simulink model "E3_2_B_Desequilibrio"  (R2018a)
settings: Solver=VariableStepAuto  StartTime=0.0  StopTime=1  RelTol=1e-3
libraries: powerlib x22, powerlib_meascontrol x20
settings Model: Creator=Rafael Pavan  LastModifiedBy=Rafael Pavan

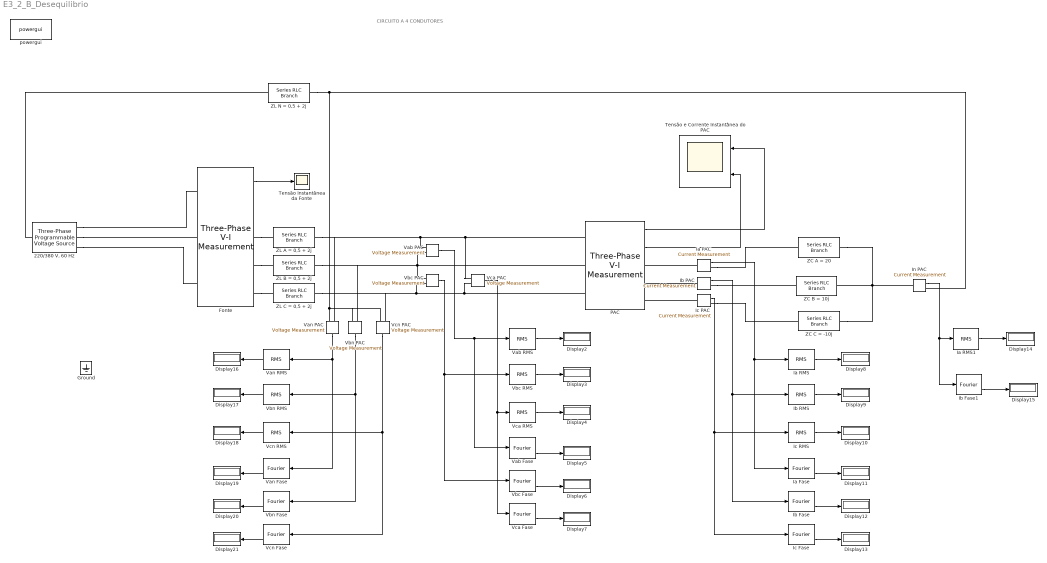
== system E3_2_B_Desequilibrio ==
  note: CIRCUITO A 4 CONDUTORES
  "220/380 V, 60 Hz" : powerlib/Electrical Sources/Three-Phase Programmable Voltage Source  PositiveSequence=[380 0 60]  VariationEntity=None  VariationType=Table of time-amplitude pairs  VariationTypeAlt=Step  VariationStep=0.5  VariationRate=10  VariationMagnitude=0.3  VariationFrequency=2  VariationTiming=[1 2]  VariationPhaseA=off  Amplitudes=[1 0.8 1.2 1.0]  TimeValues=[0 0.1 0.15 0.2]  HarmonicGeneration=off  HarmonicA=[3 0.2 -25 0]  HarmonicB=[2 0.15 35 2]  Timing="[0.05  3]"  BusType=PV  Pref=1000000000  Qref=0  Qmin=-inf  Qmax=inf
  Display{2..21} (20 alike) : Display
  Fonte : powerlib/Measurements/Three-Phase V-I Measurement  VoltageMeasurement=phase-to-phase  SetLabelV=off  LabelV=Vabc  Vpu=off  VpuLL=off  CurrentMeasurement=yes  SetLabelI=off  LabelI=Iabc  Ipu=off  Pbase=100e6  Vbase=220  OutputType=Complex  PhasorSimulation=off  PSBequivalent=0
  Ground : powerlib/Elements/Ground  LConnTagsString=a
  Ia Fase : powerlib_meascontrol/Measurements/Fourier  Freq=60  n=1  InInit=[0, 0]  Ts=0
      settings: SourceProductName=Simscape Power Systems
  Ia PAC : powerlib/Measurements/Current Measurement  PhasorSimulation=off  OutputType=Complex  PSBequivalent=0
  Ia RMS : powerlib_meascontrol/Measurements/RMS  TrueRMS=on  Freq=60  RMSInit=120  Ts=0
  Ia RMS1 : powerlib_meascontrol/Measurements/RMS  TrueRMS=on  Freq=60  RMSInit=120  Ts=0
  Ib Fase : powerlib_meascontrol/Measurements/Fourier  Freq=60  n=1  InInit=[0, 0]  Ts=0
      settings: SourceProductName=Simscape Power Systems
  Ib Fase1 : powerlib_meascontrol/Measurements/Fourier  Freq=60  n=1  InInit=[0, 0]  Ts=0
      settings: SourceProductName=Simscape Power Systems
  Ib PAC : powerlib/Measurements/Current Measurement  PhasorSimulation=off  OutputType=Complex  PSBequivalent=0
  Ib RMS : powerlib_meascontrol/Measurements/RMS  TrueRMS=on  Freq=60  RMSInit=120  Ts=0
  Ic Fase : powerlib_meascontrol/Measurements/Fourier  Freq=60  n=1  InInit=[0, 0]  Ts=0
      settings: SourceProductName=Simscape Power Systems
  Ic PAC : powerlib/Measurements/Current Measurement  PhasorSimulation=off  OutputType=Complex  PSBequivalent=0
  Ic RMS : powerlib_meascontrol/Measurements/RMS  TrueRMS=on  Freq=60  RMSInit=120  Ts=0
  In PAC : powerlib/Measurements/Current Measurement  PhasorSimulation=off  OutputType=Complex  PSBequivalent=0
  PAC : powerlib/Measurements/Three-Phase V-I Measurement  VoltageMeasurement=phase-to-phase  SetLabelV=off  LabelV=Vabc  Vpu=off  VpuLL=off  CurrentMeasurement=yes  SetLabelI=off  LabelI=Iabc  Ipu=off  Pbase=100e6  Vbase=220  OutputType=Complex  PhasorSimulation=off  PSBequivalent=0
  Tensão Instantânea da Fonte : Scope
  Tensão e Corrente Instantânea do PAC : Scope  NumInputPorts=2
  Vab Fase : powerlib_meascontrol/Measurements/Fourier  Freq=60  n=1  InInit=[0, 0]  Ts=0
      settings: SourceProductName=Simscape Power Systems
  Vab PAC : powerlib/Measurements/Voltage Measurement  PhasorSimulation=off  OutputType=Complex  PSBequivalent=0
  Vab RMS : powerlib_meascontrol/Measurements/RMS  TrueRMS=on  Freq=60  RMSInit=120  Ts=0
  Van Fase : powerlib_meascontrol/Measurements/Fourier  Freq=60  n=1  InInit=[0, 0]  Ts=0
      settings: SourceProductName=Simscape Power Systems
  Van PAC : powerlib/Measurements/Voltage Measurement  PhasorSimulation=off  OutputType=Complex  PSBequivalent=0
  Van RMS : powerlib_meascontrol/Measurements/RMS  TrueRMS=on  Freq=60  RMSInit=120  Ts=0
  Vbc Fase : powerlib_meascontrol/Measurements/Fourier  Freq=60  n=1  InInit=[0, 0]  Ts=0
      settings: SourceProductName=Simscape Power Systems
  Vbc PAC : powerlib/Measurements/Voltage Measurement  PhasorSimulation=off  OutputType=Complex  PSBequivalent=0
  Vbc RMS : powerlib_meascontrol/Measurements/RMS  TrueRMS=on  Freq=60  RMSInit=120  Ts=0
  Vbn Fase : powerlib_meascontrol/Measurements/Fourier  Freq=60  n=1  InInit=[0, 0]  Ts=0
      settings: SourceProductName=Simscape Power Systems
  Vbn PAC : powerlib/Measurements/Voltage Measurement  PhasorSimulation=off  OutputType=Complex  PSBequivalent=0
  Vbn RMS : powerlib_meascontrol/Measurements/RMS  TrueRMS=on  Freq=60  RMSInit=120  Ts=0
  Vca Fase : powerlib_meascontrol/Measurements/Fourier  Freq=60  n=1  InInit=[0, 0]  Ts=0
      settings: SourceProductName=Simscape Power Systems
  Vca PAC : powerlib/Measurements/Voltage Measurement  PhasorSimulation=off  OutputType=Complex  PSBequivalent=0
  Vca RMS : powerlib_meascontrol/Measurements/RMS  TrueRMS=on  Freq=60  RMSInit=120  Ts=0
  Vcn Fase : powerlib_meascontrol/Measurements/Fourier  Freq=60  n=1  InInit=[0, 0]  Ts=0
      settings: SourceProductName=Simscape Power Systems
  Vcn PAC : powerlib/Measurements/Voltage Measurement  PhasorSimulation=off  OutputType=Complex  PSBequivalent=0
  Vcn RMS : powerlib_meascontrol/Measurements/RMS  TrueRMS=on  Freq=60  RMSInit=120  Ts=0
  ZC A = 20 : powerlib/Elements/Series RLC Branch  LConnTagsString=__new0  RConnTagsString=__new0  BranchType=R  Resistance=20  Inductance=0  SetiL0=off  InitialCurrent=0  Capacitance=1e-6  Setx0=off  InitialVoltage=0  Measurements=None
  ZC B = 10j : powerlib/Elements/Series RLC Branch  LConnTagsString=__new0  RConnTagsString=__new0  BranchType=L  Resistance=0  Inductance=26.525e-3  SetiL0=off  InitialCurrent=0  Capacitance=1e-6  Setx0=off  InitialVoltage=0  Measurements=None
  ZC C = -10j : powerlib/Elements/Series RLC Branch  LConnTagsString=__new0  RConnTagsString=__new0  BranchType=C  Resistance=0.5  Inductance=2.65266e-4  SetiL0=off  InitialCurrent=0  Capacitance=2.652660619e-4  Setx0=off  InitialVoltage=0  Measurements=None
  ZL A = 0,5 + 2j : powerlib/Elements/Series RLC Branch  LConnTagsString=__new0  RConnTagsString=__new0  BranchType=RL  Resistance=0.5  Inductance=5.305e-3  SetiL0=off  InitialCurrent=0  Capacitance=1e-6  Setx0=off  InitialVoltage=0  Measurements=None
  ZL B = 0,5 + 2j : powerlib/Elements/Series RLC Branch  LConnTagsString=__new0  RConnTagsString=__new0  BranchType=RL  Resistance=0.5  Inductance=5.305e-3  SetiL0=off  InitialCurrent=0  Capacitance=1e-6  Setx0=off  InitialVoltage=0  Measurements=None
  ZL C = 0,5 + 2j : powerlib/Elements/Series RLC Branch  LConnTagsString=__new0  RConnTagsString=__new0  BranchType=RL  Resistance=0.5  Inductance=5.305e-3  SetiL0=off  InitialCurrent=0  Capacitance=1e-6  Setx0=off  InitialVoltage=0  Measurements=None
  "ZL N = 0,5 + 2j " : powerlib/Elements/Series RLC Branch  LConnTagsString=__new0  RConnTagsString=__new0  BranchType=RL  Resistance=0.5  Inductance=5.305e-3  SetiL0=off  InitialCurrent=0  Capacitance=1e-6  Setx0=off  InitialVoltage=0  Measurements=None
  powergui : powerlib/powergui  Priority=1  SimulationMode=Continuous  SampleTime=50e-6  frequency=60  Iterations=50  frequencyindice=60  Pbase=100e6  ErrMax=1e-4  UnitsV=kV  UnitsW=MW  buscounter=0  FunctionMessages=on  echomessages=off  EnableUseOfTLC=off  CurrentSourceSwitches=off  DisableSnubberDevices=off  DisableRonSwitches=off  DisableVfSwitches=off  DisplayEquations=off  SolverType=Tustin/Backward Euler (TBE)  Interpol=off  ExternalGateDelay=off  methode=off  Ts=100  x0status=blocks  SPID=on  SwTol=0  HookPort=off  RestoreLinks=warning  ResistiveCurrentMeasurement=off  Frange=[0:2:500]  Ylog=off  Xlog=on  ShowGrid=off  save=off  variable=ZData  structure=0  ZoomFFT=off  StartTime=0.0  cycles=1  DisplayStyle=1  fundamental=60  FreqAxis=off  MaxFrequency=1000  frequencyindicesteady=1  RmsSteady=2  display=off
  wires:
  PAC/1 -> Tensão e Corrente Instantânea do PAC/1
  Vab RMS/1 -> Display2/1
  Vbc RMS/1 -> Display3/1
  Vca RMS/1 -> Display4/1
  Vbc PAC/1 -> Vbc RMS/1, Vbc Fase/1
  Vca PAC/1 -> Vca Fase/1, Vca RMS/1
  Vab PAC/1 -> Vab Fase/1, Vab RMS/1
  Vca Fase/2 -> Display7/1
  Vab Fase/2 -> Display5/1
  Vbc Fase/2 -> Display6/1
  Ia Fase/2 -> Display11/1
  Ic RMS/1 -> Display10/1
  Ia RMS/1 -> Display8/1
  Ib Fase/2 -> Display12/1
  Ib RMS/1 -> Display9/1
  Ia PAC/1 -> Ia RMS/1, Ia Fase/1
  Ib PAC/1 -> Ib RMS/1, Ib Fase/1
  Ic PAC/1 -> Ic RMS/1, Ic Fase/1
  Ic Fase/2 -> Display13/1
  Fonte/1 -> Tensão Instantânea da Fonte/1
  In PAC/1 -> Ia RMS1/1, Ib Fase1/1
  Ia RMS1/1 -> Display14/1
  Ib Fase1/2 -> Display15/1
  Van Fase/2 -> Display19/1
  Vcn Fase/2 -> Display21/1
  Vcn RMS/1 -> Display18/1
  Van RMS/1 -> Display16/1
  Vbn Fase/2 -> Display20/1
  Vbn RMS/1 -> Display17/1
  Van PAC/1 -> Van Fase/1, Van RMS/1
  Vbn PAC/1 -> Vbn RMS/1, Vbn Fase/1
  Vcn PAC/1 -> Vcn Fase/1, Vcn RMS/1
  PAC/2 -> Tensão e Corrente Instantânea do PAC/2
  connections:
  PAC/LConn3 -- Vcn PAC/LConn1 -- ZL C = 0,5 + 2j/RConn1 -- Vbc PAC/LConn2 -- Vca PAC/LConn1
  ZC A = 20/RConn1 -- In PAC/LConn1 -- ZC C = -10j/RConn1 -- ZC B = 10j/RConn1
  PAC/LConn2 -- Vbn PAC/LConn1 -- ZL B = 0,5 + 2j/RConn1 -- Vbc PAC/LConn1 -- Vab PAC/LConn2
  PAC/LConn1 -- Van PAC/LConn1 -- ZL A = 0,5 + 2j/RConn1 -- Vab PAC/LConn1 -- Vca PAC/LConn2
  Ia PAC/LConn1 -- PAC/RConn1
  Ia PAC/RConn1 -- ZC A = 20/LConn1
  Ib PAC/LConn1 -- PAC/RConn2
  Ib PAC/RConn1 -- ZC B = 10j/LConn1
  Ic PAC/LConn1 -- PAC/RConn3
  Ic PAC/RConn1 -- ZC C = -10j/LConn1
  "220/380 V, 60 Hz"/RConn2 -- Fonte/LConn2
  "220/380 V, 60 Hz"/RConn3 -- Fonte/LConn3
  "220/380 V, 60 Hz"/RConn1 -- Fonte/LConn1
  Fonte/RConn1 -- ZL A = 0,5 + 2j/LConn1
  Fonte/RConn2 -- ZL B = 0,5 + 2j/LConn1
  Fonte/RConn3 -- ZL C = 0,5 + 2j/LConn1
  "220/380 V, 60 Hz"/LConn1 -- "ZL N = 0,5 + 2j "/LConn1
  "ZL N = 0,5 + 2j "/RConn1 -- Vcn PAC/LConn2 -- Vbn PAC/LConn2 -- Van PAC/LConn2 -- In PAC/RConn1
